simulink model "Auto_sintonizable_FuzziPID"  (R2021a)
settings: Solver=VariableStepAuto  StartTime=0.0  StopTime=10.0  RelTol=1e-3
libraries: fuzblock x8
settings Model: Creator=Nestor  LastModifiedBy=Nestor

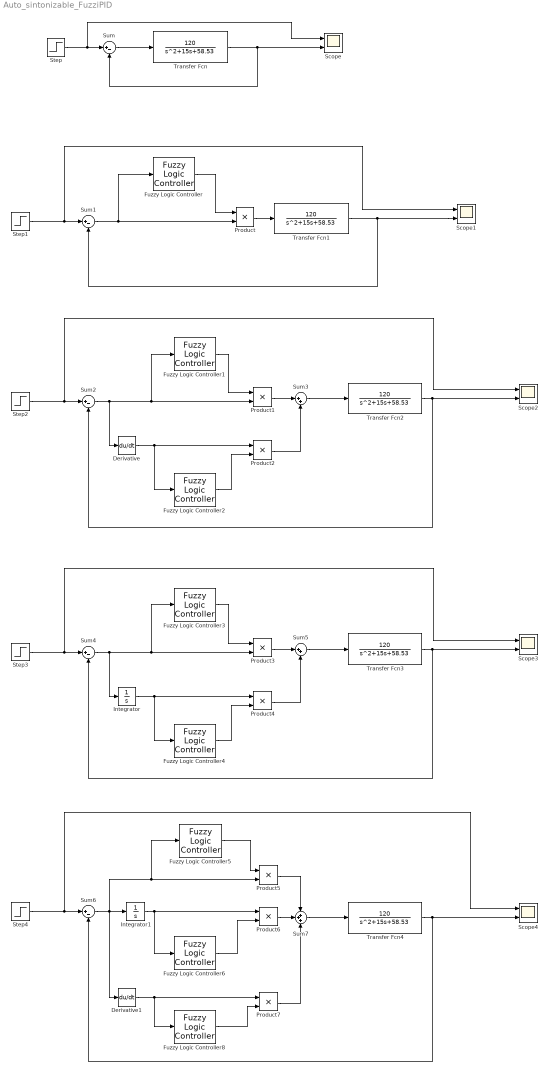
== system Auto_sintonizable_FuzziPID ==
  Derivative : Derivative
  Derivative1 : Derivative
  Fuzzy Logic Controller{,1,3,5} (4 alike) : fuzblock/Fuzzy Logic  Controller  FIS=sintoniaKp  OutputSampleNumber=101  DataType=double  FuzzifiedInputs=off  RuleFiringStrengths=off  RuleOutputs=off  AggregatedOutputs=off  SimulateUsing=Interpreted execution  OutOfRangeInputValueMessage=warning  NoRuleFiredMessage=warning  EmptyOutputFuzzySetMessage=warning
  Fuzzy Logic Controller2 : fuzblock/Fuzzy Logic  Controller  FIS=sintoniaKd  OutputSampleNumber=101  DataType=double  FuzzifiedInputs=off  RuleFiringStrengths=off  RuleOutputs=off  AggregatedOutputs=off  SimulateUsing=Interpreted execution  OutOfRangeInputValueMessage=warning  NoRuleFiredMessage=warning  EmptyOutputFuzzySetMessage=warning
  Fuzzy Logic Controller4 : fuzblock/Fuzzy Logic  Controller  FIS=sintoniaKi  OutputSampleNumber=101  DataType=double  FuzzifiedInputs=off  RuleFiringStrengths=off  RuleOutputs=off  AggregatedOutputs=off  SimulateUsing=Interpreted execution  OutOfRangeInputValueMessage=warning  NoRuleFiredMessage=warning  EmptyOutputFuzzySetMessage=warning
  Fuzzy Logic Controller6 : fuzblock/Fuzzy Logic  Controller  FIS=sintoniaKi  OutputSampleNumber=101  DataType=double  FuzzifiedInputs=off  RuleFiringStrengths=off  RuleOutputs=off  AggregatedOutputs=off  SimulateUsing=Interpreted execution  OutOfRangeInputValueMessage=warning  NoRuleFiredMessage=warning  EmptyOutputFuzzySetMessage=warning
  Fuzzy Logic Controller8 : fuzblock/Fuzzy Logic  Controller  FIS=sintoniaKd  OutputSampleNumber=101  DataType=double  FuzzifiedInputs=off  RuleFiringStrengths=off  RuleOutputs=off  AggregatedOutputs=off  SimulateUsing=Interpreted execution  OutOfRangeInputValueMessage=warning  NoRuleFiredMessage=warning  EmptyOutputFuzzySetMessage=warning
  Integrator : Integrator
  Integrator1 : Integrator
  Product{,1..7} (8 alike) : Product
  Scope{,1..4} (5 alike) : Scope  NumInputPorts=2
  Step : Step  SampleTime=0
  Step1 : Step  Before=1  SampleTime=0
  Step2 : Step  Before=1  SampleTime=0
  Step3 : Step  Time=0  After=3  SampleTime=0
  Step4 : Step  Time=0  SampleTime=0
  Sum{,1..2,4,6} (5 alike) : Sum  Inputs=|+-
  Sum3 : Sum  Inputs=|++
  Sum5 : Sum  Inputs=|++
  Sum7 : Sum  Inputs=+++
  Transfer Fcn{,1..4} (5 alike) : TransferFcn  Numerator=[120]  Denominator=[1 15 58.53]
  wires:
  Step/1 -> Scope/1, Sum/1
  Transfer Fcn/1 -> Sum/2, Scope/2
  Sum/1 -> Transfer Fcn/1
  Transfer Fcn1/1 -> Sum1/2, Scope1/2
  Step1/1 -> Sum1/1, Scope1/1
  Sum1/1 -> Fuzzy Logic Controller/1, Product/2
  Product/1 -> Transfer Fcn1/1
  Fuzzy Logic Controller/1 -> Product/1
  Step2/1 -> Sum2/1, Scope2/1
  Transfer Fcn2/1 -> Sum2/2, Scope2/2
  Fuzzy Logic Controller1/1 -> Product1/1
  Sum2/1 -> Derivative/1, Fuzzy Logic Controller1/1, Product1/2
  Product1/1 -> Sum3/1
  Sum3/1 -> Transfer Fcn2/1
  Derivative/1 -> Fuzzy Logic Controller2/1, Product2/1
  Fuzzy Logic Controller2/1 -> Product2/2
  Product2/1 -> Sum3/2
  Product4/1 -> Sum5/2
  Fuzzy Logic Controller4/1 -> Product4/2
  Product3/1 -> Sum5/1
  Fuzzy Logic Controller3/1 -> Product3/1
  Transfer Fcn3/1 -> Sum4/2, Scope3/2
  Step3/1 -> Sum4/1, Scope3/1
  Integrator/1 -> Fuzzy Logic Controller4/1, Product4/1
  Sum4/1 -> Integrator/1, Fuzzy Logic Controller3/1, Product3/2
  Sum5/1 -> Transfer Fcn3/1
  Transfer Fcn4/1 -> Scope4/2, Sum6/2
  Fuzzy Logic Controller6/1 -> Product6/2
  Step4/1 -> Sum6/1, Scope4/1
  Fuzzy Logic Controller5/1 -> Product5/1
  Product5/1 -> Sum7/1
  Sum7/1 -> Transfer Fcn4/1
  Product6/1 -> Sum7/2
  Integrator1/1 -> Fuzzy Logic Controller6/1, Product6/1
  Product7/1 -> Sum7/3
  Fuzzy Logic Controller8/1 -> Product7/2
  Derivative1/1 -> Fuzzy Logic Controller8/1, Product7/1
  Sum6/1 -> Derivative1/1, Integrator1/1, Fuzzy Logic Controller5/1, Product5/2
